simulink model "AGTF30SysDyn"  (R2021b)
settings: Solver=ode4  StartTime=0.0  StopTime=MWS.In.Tsim  FixedStep=MWS.In.Ts  RelTol=1e-3  EnableMultiTasking=on
model workspace: external: MAT-File (data not in the file)
undefined symbols (not defined in the file): MWS, VAFNact, VBVact
libraries: Lib_Cntrl_FirstOrderSensor_TMATS x12, Lib_Cntrl_SetPoint_TMATS x2, Lib_Solve_OuterLoopIntegrator_TMATS x2, simulink x2, Lib_Cntrl_FirstOrderActuator_TMATS x1, Lib_Cntrl_CorrectedSpeed_TMATS x1, Lib_Solve_IterNRSolverJC_TMATS x1
settings Model: Creator=jwchapm2  LastModifiedBy=prbalm
settings SolverCC: AlgebraicLoopSolver=TrustRegion
settings DataIOCC: LimitDataPoints=on  SaveFormat=Array  ReturnWorkspaceOutputs=off
settings OptimizationCC: LifeSpan=inf
settings DebuggingCC: SFUnexpectedBacktrackingDiag=warning  SFNoUnconditionalDefaultTransitionDiag=warning  SFExecutionAtInitializationDiag=none  SFMachineParentedDataDiag=warning  ArithmeticOperatorsInVariantConditions=warning
settings HardwareCC: ProdBitPerPointer=32  ProdBitPerSizeT=32  ProdBitPerPtrDiffT=32  ProdLargestAtomicFloat=None  ProdIntDivRoundTo=Undefined  ProdEndianess=Unspecified  ProdWordSize=32  ProdHWDeviceType=32-bit Generic
settings ModelReferenceCC: PropagateSignalLabelsOutOfModel=off
settings SFSimCC: SimUseLocalCustomCode=off  CustomCodeUndefinedFunction=UseInterfaceOnly
settings RTWCC: RTWUseLocalCustomCode=off
settings CodeAppCC: StateflowObjectComments=on
settings GRTTargetCC: TargetLangStandard=C89/C90 (ANSI)
settings ConfigComp: CovMetricSettings=dw  CovSaveCumulativeToWorkspaceVar=on  CovSaveSingleToWorkspaceVar=on  CovExternalEMLEnable=off

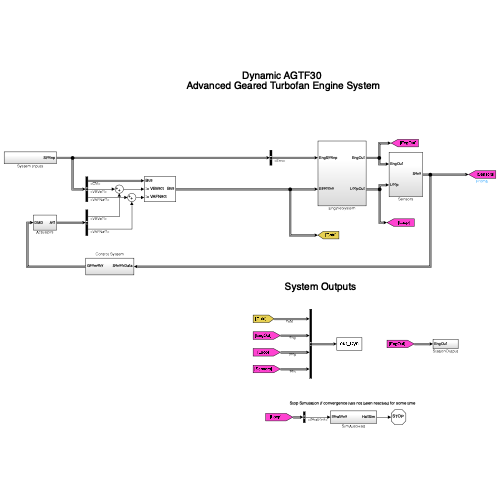
[thumbnail: Simulink's stored preview of the top-level diagram]
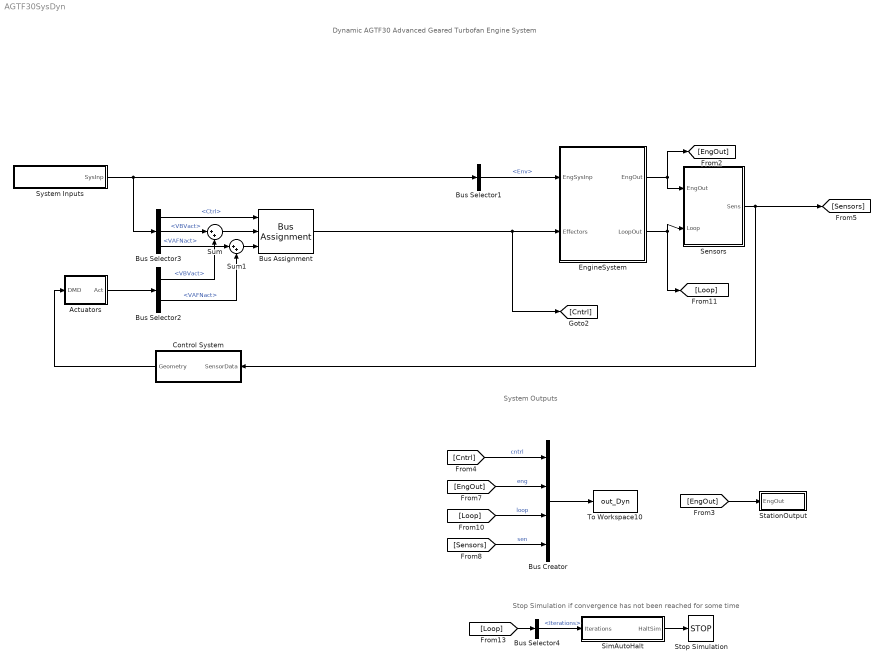
== system AGTF30SysDyn ==
  note: Stop Simulation if convergence has not been reached for some time
  note: Dynamic AGTF30
      | Advanced Geared Turbofan Engine System
  note: System Outputs
  Actuators : Subsystem
  Bus Assignment : BusAssignment  AssignedSignals=VBVact,VAFNact
  Bus Creator : BusCreator  Inputs=4
  Bus Selector1 : BusSelector  OutputSignals=Env
  Bus Selector2 : BusSelector  OutputSignals=VBVact,VAFNact
  Bus Selector3 : BusSelector  OutputSignals=Ctrl,Ctrl.VBVact,Ctrl.VAFNact
  Bus Selector4 : BusSelector  OutputSignals=Solver.Iterations
  Control System : Subsystem
  EngineSystem : Subsystem
  Sensors : Subsystem
  SimAutoHalt : Subsystem
  StationOutput : Subsystem
  Stop Simulation : Stop
  Sum : Sum  Inputs=|++
  Sum1 : Sum  Inputs=|++
  System Inputs : Subsystem
  To Workspace10 : ToWorkspace  VariableName=out_Dyn  SaveFormat=Timeseries  SampleTime=-1
  wires:
  EngineSystem/1(EngOut) -> Sensors/1(EngOut), [EngOut]
  EngineSystem/2(LoopOut) -> Sensors/2(Loop), [Loop]
  [EngOut] -> StationOutput/1(EngOut)
  Bus Creator/1 -> To Workspace10/1
  [Loop] -> Bus Creator/3  "loop"
  [Sensors] -> Bus Creator/4  "sen"
  [EngOut] -> Bus Creator/2  "eng"
  [Cntrl] -> Bus Creator/1  "cntrl"
  [Loop] -> Bus Selector4/1
  Bus Selector4/1 -> SimAutoHalt/1(Iterations)  "<Iterations>"
  SimAutoHalt/1(HaltSim) -> Stop Simulation/1
  Actuators/1(Act) -> Bus Selector2/1
  Control System/1(Geometry) -> Actuators/1(DMD)
  System Inputs/1(SysInp) -> Bus Selector1/1, Bus Selector3/1
  Bus Assignment/1 -> [Cntrl], EngineSystem/2(Effectors)
  Sensors/1(Sens) -> [Sensors], Control System/1(SensorData)
  Bus Selector3/2 -> Sum/1  "<VBVact>"
  Bus Selector2/1 -> Sum/2  "<VBVact>"
  Bus Selector2/2 -> Sum1/2  "<VAFNact>"
  Sum1/1 -> Bus Assignment/3
  Bus Selector1/1 -> EngineSystem/1(EngSysInp)  "<Env>"
  Sum/1 -> Bus Assignment/2
  Bus Selector3/3 -> Sum1/1  "<VAFNact>"
  Bus Selector3/1 -> Bus Assignment/1  "<Ctrl>"

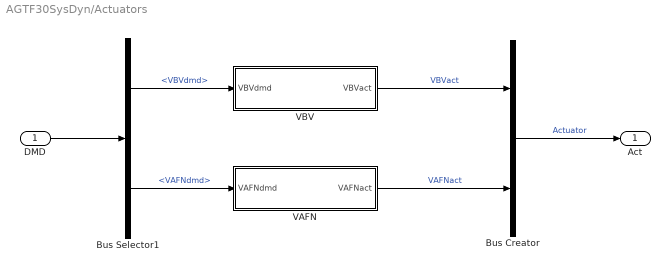
== system AGTF30SysDyn/Actuators ==
  DMD : Inport
  Bus Creator : BusCreator  Inputs=2
  Bus Selector1 : BusSelector  OutputSignals=VBVdmd,VAFNdmd
  VAFN : Subsystem
  VBV : Subsystem
  Act : Outport
  wires:
  DMD/1 -> Bus Selector1/1
  Bus Creator/1 -> Act/1  "Actuator"
  Bus Selector1/2 -> VAFN/1(VAFNdmd)  "<VAFNdmd>"
  Bus Selector1/1 -> VBV/1(VBVdmd)  "<VBVdmd>"
  VBV/1(VBVact) -> Bus Creator/1  "VBVact"
  VAFN/1(VAFNact) -> Bus Creator/2  "VAFNact"

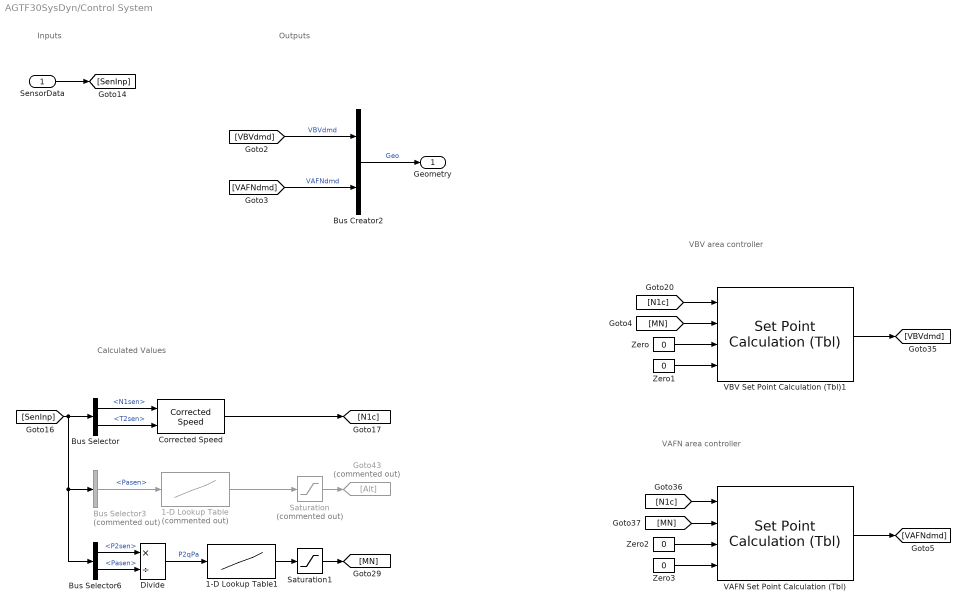
== system AGTF30SysDyn/Control System ==
  note: Inputs
  note: VAFN area controller
  note: VBV area controller
  note: Calculated Values
  note: Outputs
  SensorData : Inport
  1-D Lookup Table : Lookup_n-D  Commented=on  NumberOfTableDimensions=1  BreakpointsForDimension1=MWS.Cntrl.AltCalc_PaVec  Table=MWS.Cntrl.AltCalc_AltVec  InternalRulePriority=Speed  RndMeth=Simplest  InputSameDT=on
  1-D Lookup Table1 : Lookup_n-D  NumberOfTableDimensions=1  BreakpointsForDimension1=MWS.Cntrl.MNCalc_P2qPa  Table=MWS.Cntrl.MNCalc_MNVec  InternalRulePriority=Speed  RndMeth=Simplest  InputSameDT=on
  Bus Creator2 : BusCreator  Inputs=2
  Bus Selector : BusSelector  OutputSignals=N.N1sen,T.T2sen
  Bus Selector3 : BusSelector  Commented=on  OutputSignals=P.Pasen
  Bus Selector6 : BusSelector  OutputSignals=P.P2sen,P.Pasen
  Corrected Speed : Lib_Cntrl_CorrectedSpeed_TMATS/Corrected Speed  C_TSTD_M=518.67
  Divide : Product  Inputs=*/
  Goto43 : Goto  Commented=on  GotoTag=Alt
  Saturation : Saturate  Commented=on  UpperLimit=MWS.Cntrl.AltCalc_Altmax  LowerLimit=MWS.Cntrl.AltCalc_Altmin
  Saturation1 : Saturate  UpperLimit=MWS.Cntrl.MNCalc_MNmax  LowerLimit=MWS.Cntrl.MNCalc_MNmin
  VAFN Set Point Calculation (Tbl) : Lib_Cntrl_SetPoint_TMATS/Set Point Calculation (Tbl)  ERVec_M=MWS.Cntrl.VAFN_Nc1  DSVec_M=MWS.Cntrl.VAFN_MN  SPArray_M=MWS.Cntrl.VAFN_sch
  VBV Set Point Calculation (Tbl)1 : Lib_Cntrl_SetPoint_TMATS/Set Point Calculation (Tbl)  ERVec_M=MWS.Cntrl.VBV_Nc1  DSVec_M=MWS.Cntrl.VBV_MN  SPArray_M=MWS.Cntrl.VBV_sch
  Zero{,1..3} (4 alike) : Constant  Value=0  OutDataTypeStr=Inherit: Inherit via back propagation
  Geometry : Outport
  wires:
  [VBVdmd] -> Bus Creator2/1  "VBVdmd"
  [VAFNdmd] -> Bus Creator2/2  "VAFNdmd"
  SensorData/1 -> [SenInp]
  Bus Selector/1 -> Corrected Speed/1  "<N1sen>"
  Corrected Speed/1 -> [N1c]
  Bus Selector/2 -> Corrected Speed/2  "<T2sen>"
  VAFN Set Point Calculation (Tbl)/1 -> [VAFNdmd]
  [MN] -> VBV Set Point Calculation (Tbl)1/2
  VBV Set Point Calculation (Tbl)1/1 -> [VBVdmd]
  [MN] -> VAFN Set Point Calculation (Tbl)/2
  [N1c] -> VAFN Set Point Calculation (Tbl)/1
  [N1c] -> VBV Set Point Calculation (Tbl)1/1
  1-D Lookup Table/1 -> Saturation/1
  [SenInp] -> Bus Selector6/1, Bus Selector3/1, Bus Selector/1
  Bus Selector3/1 -> 1-D Lookup Table/1  "<Pasen>"
  Bus Selector6/1 -> Divide/1  "<P2sen>"
  Bus Selector6/2 -> Divide/2  "<Pasen>"
  Divide/1 -> 1-D Lookup Table1/1  "P2qPa"
  1-D Lookup Table1/1 -> Saturation1/1
  Saturation/1 -> Goto43/1
  Saturation1/1 -> [MN]
  Bus Creator2/1 -> Geometry/1  "Geo"
  Zero/1 -> VBV Set Point Calculation (Tbl)1/3
  Zero1/1 -> VBV Set Point Calculation (Tbl)1/4
  Zero2/1 -> VAFN Set Point Calculation (Tbl)/3
  Zero3/1 -> VAFN Set Point Calculation (Tbl)/4

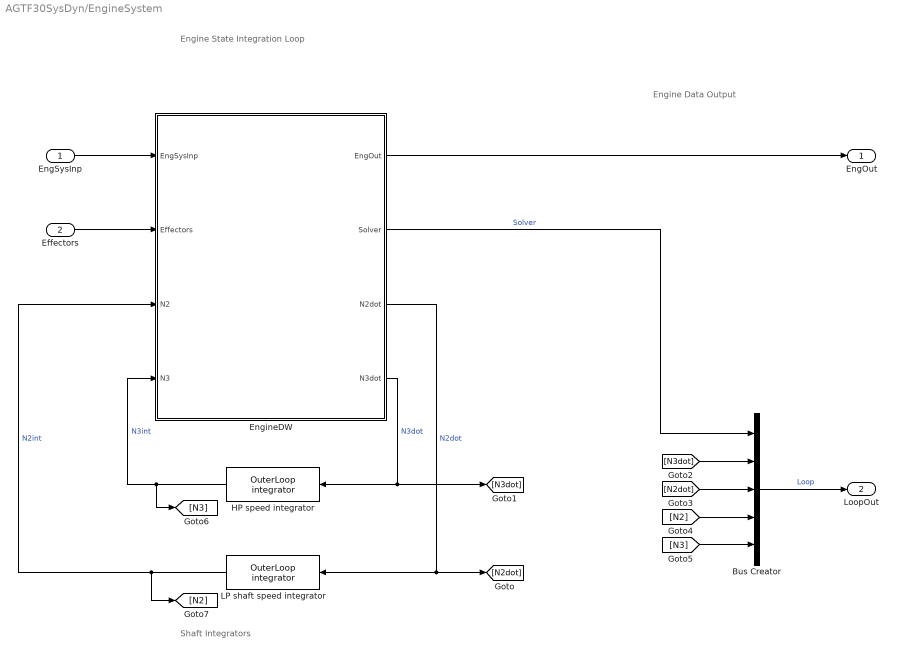
== system AGTF30SysDyn/EngineSystem ==
  note: Shaft Integrators
  note: Engine State
      | Integration Loop
  note: Engine Data Output
  EngSysInp : Inport
  Effectors : Inport  Port=2
  Bus Creator : BusCreator  Inputs=5
  EngineDW : Subsystem
  HP speed integrator : Lib_Solve_OuterLoopIntegrator_TMATS/OuterLoop integrator  OL_IC_M=MWS.In.N3IC
  LP shaft speed integrator : Lib_Solve_OuterLoopIntegrator_TMATS/OuterLoop integrator  OL_IC_M=MWS.In.N2IC
  EngOut : Outport
  LoopOut : Outport  Port=2
  wires:
  EngSysInp/1 -> EngineDW/1(EngSysInp)
  LP shaft speed integrator/1 -> [N2], EngineDW/3(N2)  "N2int"
  Effectors/1 -> EngineDW/2(Effectors)
  EngineDW/3(N2dot) -> LP shaft speed integrator/1, [N2dot]  "N2dot"
  EngineDW/2(Solver) -> Bus Creator/1  "Solver"
  EngineDW/1(EngOut) -> EngOut/1
  EngineDW/4(N3dot) -> HP speed integrator/1, [N3dot]  "N3dot"
  HP speed integrator/1 -> [N3], EngineDW/4(N3)  "N3int"
  Bus Creator/1 -> LoopOut/1  "Loop"
  [N3dot] -> Bus Creator/2
  [N2dot] -> Bus Creator/3
  [N2] -> Bus Creator/4
  [N3] -> Bus Creator/5

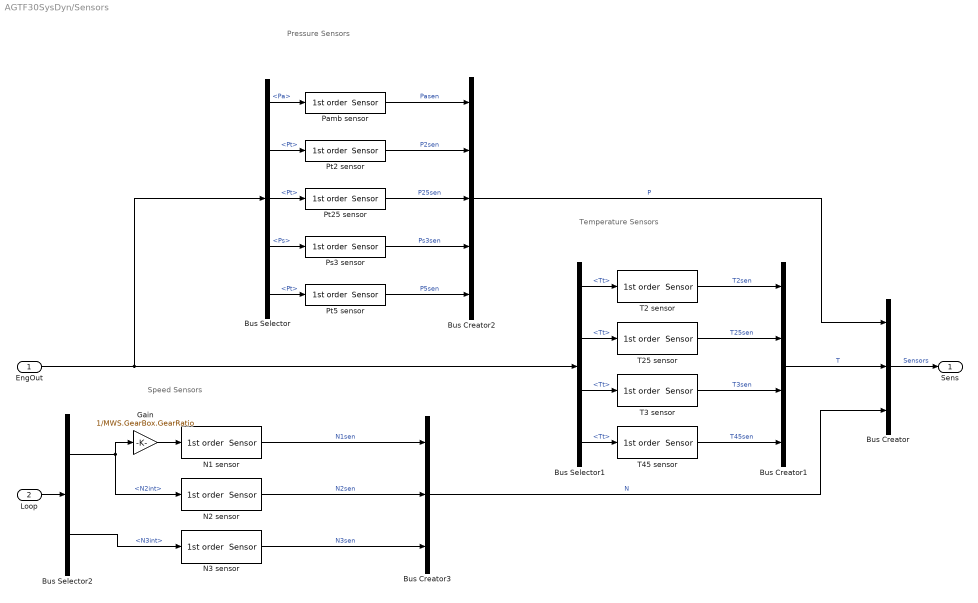
== system AGTF30SysDyn/Sensors ==
  note: Pressure Sensors
  note: Temperature Sensors
  note: Speed Sensors
  EngOut : Inport
  Loop : Inport  Port=2
  Bus Creator : BusCreator  Inputs=3
  Bus Creator1 : BusCreator  Inputs=4
  Bus Creator2 : BusCreator  Inputs=5
  Bus Creator3 : BusCreator  Inputs=3
  Bus Selector : BusSelector  OutputSignals=Amb.Pa,S2.Pt,S25.Pt,S36.Ps,S5.Pt
  Bus Selector1 : BusSelector  OutputSignals=S2.Tt,S25.Tt,S36.Tt,S45.Tt
  Bus Selector2 : BusSelector  OutputSignals=N2int,N3int
  Gain : Gain  Gain=1/MWS.GearBox.GearRatio
  N1 sensor : Lib_Cntrl_FirstOrderSensor_TMATS/1st order  Sensor  IC_M=MWS.In.Sensor.ICN1  Sen_Max_M=MWS.Sensor.N1.Max  Sen_Min_M=MWS.Sensor.N1.Min  Gain_M=1  Tau_M=MWS.Sensor.N1.Tau  GN_EN_M=off  GN_NST_M=MWS.In.Ts  GN_C_M=1  GN_MinNoise_M=0.3  F_Gain_M=1  F_Drift_M=0
  N2 sensor : Lib_Cntrl_FirstOrderSensor_TMATS/1st order  Sensor  IC_M=MWS.In.Sensor.ICN2  Sen_Max_M=MWS.Sensor.N2.Max  Sen_Min_M=MWS.Sensor.N2.Min  Gain_M=1  Tau_M=MWS.Sensor.N2.Tau  GN_EN_M=off  GN_NST_M=MWS.In.Ts  GN_C_M=1  GN_MinNoise_M=0.3  F_Gain_M=1  F_Drift_M=0
  N3 sensor : Lib_Cntrl_FirstOrderSensor_TMATS/1st order  Sensor  IC_M=MWS.In.Sensor.ICN3  Sen_Max_M=MWS.Sensor.N3.Max  Sen_Min_M=MWS.Sensor.N3.Min  Gain_M=1  Tau_M=MWS.Sensor.N3.Tau  GN_EN_M=off  GN_NST_M=MWS.In.Ts  GN_C_M=1  GN_MinNoise_M=0.3  F_Gain_M=1  F_Drift_M=0
  Pamb sensor : Lib_Cntrl_FirstOrderSensor_TMATS/1st order  Sensor  IC_M=MWS.In.Sensor.ICPa  Sen_Max_M=MWS.Sensor.P2.Max  Sen_Min_M=MWS.Sensor.P2.Min  Gain_M=1  Tau_M=MWS.Sensor.P2.Tau  GN_EN_M=off  GN_NST_M=MWS.In.Ts  GN_C_M=1  GN_MinNoise_M=0.3  F_Gain_M=1  F_Drift_M=0
  Ps3 sensor : Lib_Cntrl_FirstOrderSensor_TMATS/1st order  Sensor  IC_M=MWS.In.Sensor.ICPs3  Sen_Max_M=MWS.Sensor.Ps3.Max  Sen_Min_M=MWS.Sensor.Ps3.Min  Gain_M=1  Tau_M=MWS.Sensor.Ps3.Tau  GN_EN_M=off  GN_NST_M=MWS.In.Ts  GN_C_M=1  GN_MinNoise_M=0.3  F_Gain_M=1  F_Drift_M=0
  Pt2 sensor : Lib_Cntrl_FirstOrderSensor_TMATS/1st order  Sensor  IC_M=MWS.In.Sensor.ICP2  Sen_Max_M=MWS.Sensor.P2.Max  Sen_Min_M=MWS.Sensor.P2.Min  Gain_M=1  Tau_M=MWS.Sensor.P2.Tau  GN_EN_M=off  GN_NST_M=MWS.In.Ts  GN_C_M=1  GN_MinNoise_M=0.3  F_Gain_M=1  F_Drift_M=0
  Pt25 sensor : Lib_Cntrl_FirstOrderSensor_TMATS/1st order  Sensor  IC_M=MWS.In.Sensor.ICP25  Sen_Max_M=MWS.Sensor.P25.Max  Sen_Min_M=MWS.Sensor.P25.Min  Gain_M=1  Tau_M=MWS.Sensor.P25.Tau  GN_EN_M=off  GN_NST_M=MWS.In.Ts  GN_C_M=1  GN_MinNoise_M=0.3  F_Gain_M=1  F_Drift_M=0
  Pt5 sensor : Lib_Cntrl_FirstOrderSensor_TMATS/1st order  Sensor  IC_M=MWS.In.Sensor.ICP5  Sen_Max_M=MWS.Sensor.P5.Max  Sen_Min_M=MWS.Sensor.P5.Min  Gain_M=1  Tau_M=MWS.Sensor.P5.Tau  GN_EN_M=off  GN_NST_M=MWS.In.Ts  GN_C_M=1  GN_MinNoise_M=0.3  F_Gain_M=1  F_Drift_M=0
  T2 sensor : Lib_Cntrl_FirstOrderSensor_TMATS/1st order  Sensor  IC_M=MWS.In.Sensor.ICT2  Sen_Max_M=MWS.Sensor.T2.Max  Sen_Min_M=MWS.Sensor.T2.Min  Gain_M=1  Tau_M=MWS.Sensor.T2.Tau  GN_EN_M=off  GN_NST_M=MWS.In.Ts  GN_C_M=1  GN_MinNoise_M=0.3  F_Gain_M=1  F_Drift_M=0
  T25 sensor : Lib_Cntrl_FirstOrderSensor_TMATS/1st order  Sensor  IC_M=MWS.In.Sensor.ICT25  Sen_Max_M=MWS.Sensor.T25.Max  Sen_Min_M=MWS.Sensor.T25.Min  Gain_M=1  Tau_M=MWS.Sensor.T25.Tau  GN_EN_M=off  GN_NST_M=MWS.In.Ts  GN_C_M=1  GN_MinNoise_M=0.3  F_Gain_M=1  F_Drift_M=0
  T3 sensor : Lib_Cntrl_FirstOrderSensor_TMATS/1st order  Sensor  IC_M=MWS.In.Sensor.ICT3  Sen_Max_M=MWS.Sensor.T3.Max  Sen_Min_M=MWS.Sensor.T3.Min  Gain_M=1  Tau_M=MWS.Sensor.T3.Tau  GN_EN_M=off  GN_NST_M=MWS.In.Ts  GN_C_M=1  GN_MinNoise_M=0.3  F_Gain_M=1  F_Drift_M=0
  T45 sensor : Lib_Cntrl_FirstOrderSensor_TMATS/1st order  Sensor  IC_M=MWS.In.Sensor.ICT45  Sen_Max_M=MWS.Sensor.T45.Max*10  Sen_Min_M=MWS.Sensor.T45.Min  Gain_M=1  Tau_M=MWS.Sensor.T45.Tau  GN_EN_M=off  GN_NST_M=MWS.In.Ts  GN_C_M=1  GN_MinNoise_M=0.3  F_Gain_M=1  F_Drift_M=0
  Sens : Outport
  wires:
  Bus Creator/1 -> Sens/1  "Sensors"
  Bus Selector/2 -> Pt2 sensor/1  "<Pt>"
  Bus Creator2/1 -> Bus Creator/1  "P"
  Bus Creator1/1 -> Bus Creator/2  "T"
  Bus Selector1/1 -> T2 sensor/1  "<Tt>"
  Bus Creator3/1 -> Bus Creator/3  "N"
  Bus Selector/3 -> Pt25 sensor/1  "<Pt>"
  Bus Selector/5 -> Pt5 sensor/1  "<Pt>"
  Pt2 sensor/1 -> Bus Creator2/2  "P2sen"
  Pt25 sensor/1 -> Bus Creator2/3  "P25sen"
  Pt5 sensor/1 -> Bus Creator2/5  "P5sen"
  Bus Selector1/2 -> T25 sensor/1  "<Tt>"
  Bus Selector1/3 -> T3 sensor/1  "<Tt>"
  Bus Selector1/4 -> T45 sensor/1  "<Tt>"
  T2 sensor/1 -> Bus Creator1/1  "T2sen"
  T25 sensor/1 -> Bus Creator1/2  "T25sen"
  T3 sensor/1 -> Bus Creator1/3  "T3sen"
  N1 sensor/1 -> Bus Creator3/1  "N1sen"
  Bus Selector/4 -> Ps3 sensor/1  "<Ps>"
  N3 sensor/1 -> Bus Creator3/3  "N3sen"
  Bus Selector/1 -> Pamb sensor/1  "<Pa>"
  Pamb sensor/1 -> Bus Creator2/1  "Pasen"
  N2 sensor/1 -> Bus Creator3/2  "N2sen"
  EngOut/1 -> Bus Selector/1, Bus Selector1/1
  Bus Selector2/2 -> N3 sensor/1  "<N3int>"
  Bus Selector2/1 -> N2 sensor/1, Gain/1  "<N2int>"
  Gain/1 -> N1 sensor/1
  Loop/1 -> Bus Selector2/1
  T45 sensor/1 -> Bus Creator1/4  "T45sen"
  Ps3 sensor/1 -> Bus Creator2/4  "Ps3sen"

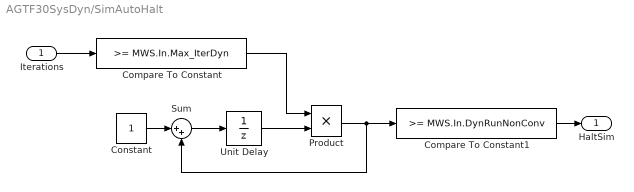
== system AGTF30SysDyn/SimAutoHalt ==
  Iterations : Inport
  Compare To Constant : simulink/Logic and Bit Operations/Compare To Constant  relop=>=  const=MWS.In.Max_IterDyn  OutDataTypeStr=boolean
  Compare To Constant1 : simulink/Logic and Bit Operations/Compare To Constant  relop=>=  const=MWS.In.DynRunNonConv  OutDataTypeStr=boolean
  Constant : Constant
  Product : Product
  Sum : Sum  Inputs=|++
  Unit Delay : UnitDelay  SampleTime=-1  HasFrameUpgradeWarning=on
  HaltSim : Outport
  wires:
  Compare To Constant1/1 -> HaltSim/1
  Iterations/1 -> Compare To Constant/1
  Compare To Constant/1 -> Product/1
  Constant/1 -> Sum/1
  Sum/1 -> Unit Delay/1
  Unit Delay/1 -> Product/2
  Product/1 -> Sum/2, Compare To Constant1/1

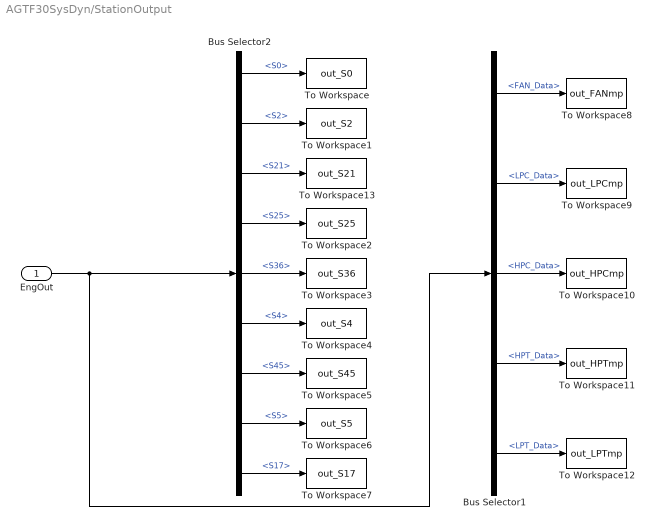
== system AGTF30SysDyn/StationOutput ==
  EngOut : Inport
  Bus Selector1 : BusSelector  OutputSignals=Data.FAN_Data,Data.LPC_Data,Data.HPC_Data,Data.HPT_Data,Data.LPT_Data
  Bus Selector2 : BusSelector  OutputSignals=S0,S2,S21,S25,S36,S4,S45,S5,S17
  To Workspace : ToWorkspace  VariableName=out_S0  SaveFormat=Timeseries  SampleTime=-1
  To Workspace1 : ToWorkspace  VariableName=out_S2  SaveFormat=Timeseries  SampleTime=-1
  To Workspace10 : ToWorkspace  VariableName=out_HPCmp  SaveFormat=Timeseries  SampleTime=-1
  To Workspace11 : ToWorkspace  VariableName=out_HPTmp  SaveFormat=Timeseries  SampleTime=-1
  To Workspace12 : ToWorkspace  VariableName=out_LPTmp  SaveFormat=Timeseries  SampleTime=-1
  To Workspace13 : ToWorkspace  VariableName=out_S21  SaveFormat=Timeseries  SampleTime=-1
  To Workspace2 : ToWorkspace  VariableName=out_S25  SaveFormat=Timeseries  SampleTime=-1
  To Workspace3 : ToWorkspace  VariableName=out_S36  SaveFormat=Timeseries  SampleTime=-1
  To Workspace4 : ToWorkspace  VariableName=out_S4  SaveFormat=Timeseries  SampleTime=-1
  To Workspace5 : ToWorkspace  VariableName=out_S45  SaveFormat=Timeseries  SampleTime=-1
  To Workspace6 : ToWorkspace  VariableName=out_S5  SaveFormat=Timeseries  SampleTime=-1
  To Workspace7 : ToWorkspace  VariableName=out_S17  SaveFormat=Timeseries  SampleTime=-1
  To Workspace8 : ToWorkspace  VariableName=out_FANmp  SaveFormat=Timeseries  SampleTime=-1
  To Workspace9 : ToWorkspace  VariableName=out_LPCmp  SaveFormat=Timeseries  SampleTime=-1
  wires:
  Bus Selector2/3 -> To Workspace13/1  "<S21>"
  Bus Selector2/1 -> To Workspace/1  "<S0>"
  EngOut/1 -> Bus Selector1/1, Bus Selector2/1
  Bus Selector2/2 -> To Workspace1/1  "<S2>"
  Bus Selector2/4 -> To Workspace2/1  "<S25>"
  Bus Selector2/5 -> To Workspace3/1  "<S36>"
  Bus Selector2/6 -> To Workspace4/1  "<S4>"
  Bus Selector2/7 -> To Workspace5/1  "<S45>"
  Bus Selector2/8 -> To Workspace6/1  "<S5>"
  Bus Selector2/9 -> To Workspace7/1  "<S17>"
  Bus Selector1/1 -> To Workspace8/1  "<FAN_Data>"
  Bus Selector1/2 -> To Workspace9/1  "<LPC_Data>"
  Bus Selector1/3 -> To Workspace10/1  "<HPC_Data>"
  Bus Selector1/4 -> To Workspace11/1  "<HPT_Data>"
  Bus Selector1/5 -> To Workspace12/1  "<LPT_Data>"

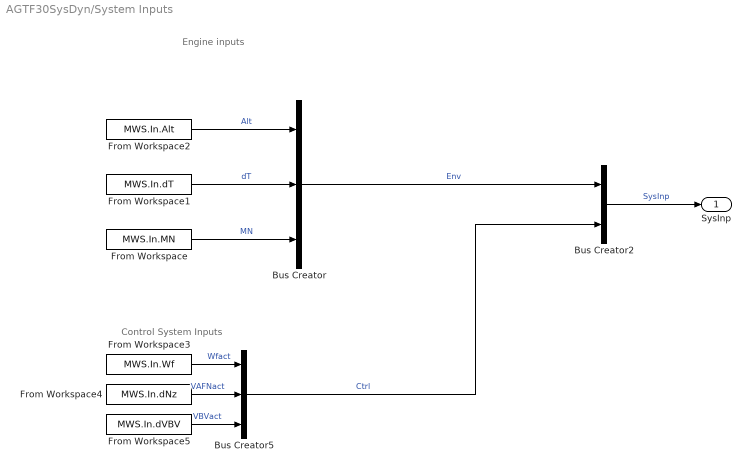
== system AGTF30SysDyn/System Inputs ==
  note: Engine inputs
  note: Control System Inputs
  Bus Creator : BusCreator  Inputs=3
  Bus Creator2 : BusCreator  Inputs=2
  Bus Creator5 : BusCreator  Inputs=3
  From Workspace : FromWorkspace  VariableName=MWS.In.MN
  From Workspace1 : FromWorkspace  VariableName=MWS.In.dT
  From Workspace2 : FromWorkspace  VariableName=MWS.In.Alt
  From Workspace3 : FromWorkspace  VariableName=MWS.In.Wf
  From Workspace4 : FromWorkspace  VariableName=MWS.In.dNz
  From Workspace5 : FromWorkspace  VariableName=MWS.In.dVBV
  SysInp : Outport
  wires:
  From Workspace2/1 -> Bus Creator/1  "Alt"
  From Workspace1/1 -> Bus Creator/2  "dT"
  From Workspace/1 -> Bus Creator/3  "MN"
  Bus Creator/1 -> Bus Creator2/1  "Env"
  Bus Creator5/1 -> Bus Creator2/2  "Ctrl"
  Bus Creator2/1 -> SysInp/1  "SysInp"
  From Workspace3/1 -> Bus Creator5/1  "Wfact"
  From Workspace4/1 -> Bus Creator5/2  "VAFNact"
  From Workspace5/1 -> Bus Creator5/3  "VBVact"

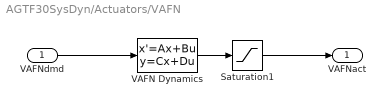
== system AGTF30SysDyn/Actuators/VAFN ==
  VAFNdmd : Inport
  Saturation1 : Saturate  UpperLimit=MWS.Act.VAFN_max  LowerLimit=0  LinearizeAsGain=off
  VAFN Dynamics : StateSpace  A=MWS.Act.VAFN.A  B=MWS.Act.VAFN.B  C=MWS.Act.VAFN.C  D=MWS.Act.VAFN.D  InitialCondition=MWS.In.VAFNIC
  VAFNact : Outport
  wires:
  Saturation1/1 -> VAFNact/1
  VAFNdmd/1 -> VAFN Dynamics/1
  VAFN Dynamics/1 -> Saturation1/1

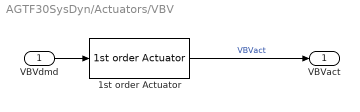
== system AGTF30SysDyn/Actuators/VBV ==
  VBVdmd : Inport
  1st order Actuator : Lib_Cntrl_FirstOrderActuator_TMATS/1st order Actuator  Gain_M=MWS.Act.VBV.Gain  Tau_M=MWS.Act.VBV.Tau  IC_M=MWS.In.VBVIC  MaxSat_M=MWS.Act.VBV.max  MinSat_M=MWS.Act.VBV.min  deadband_M=0.0  rateLimit_M=100000
  VBVact : Outport
  wires:
  VBVdmd/1 -> 1st order Actuator/1
  1st order Actuator/1 -> VBVact/1  "VBVact"

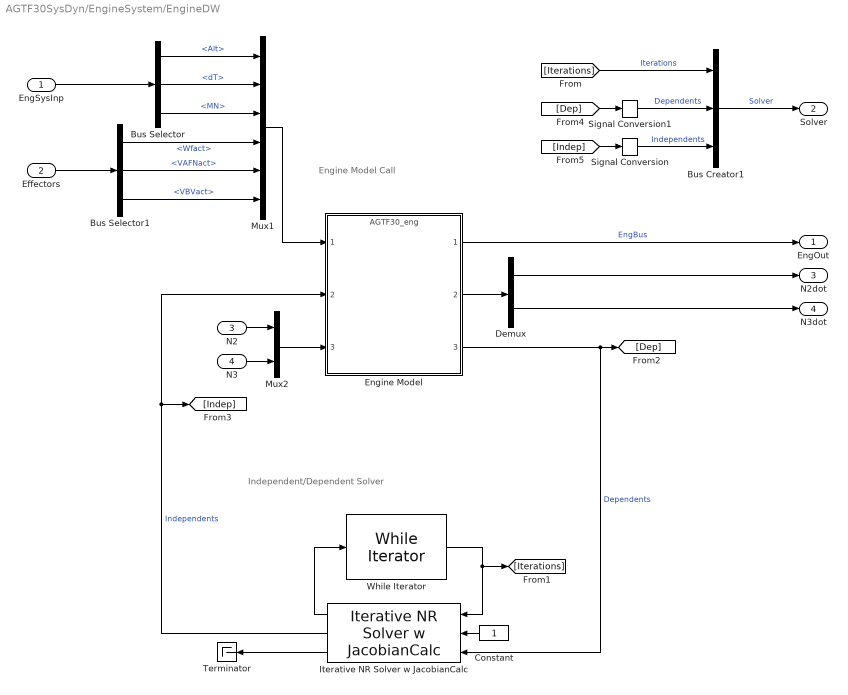
== system AGTF30SysDyn/EngineSystem/EngineDW ==
  note: Independent/Dependent Solver
  note: Engine Model Call
  EngSysInp : Inport
  Effectors : Inport  Port=2
  N2 : Inport  Port=3
  N3 : Inport  Port=4
  Bus Creator1 : BusCreator  Inputs=3
  Bus Selector : BusSelector  OutputSignals=Alt,dT,MN
  Bus Selector1 : BusSelector  OutputSignals=Wfact,VAFNact,VBVact
  Constant : Constant
  Demux : Demux  Outputs=2
  Engine Model : ModelReference  ModelNameDialog=AGTF30_eng.mdl  SimulationMode=Normal  ModelReferenceVersion=1.306
  Iterative NR Solver w JacobianCalc : Lib_Solve_IterNRSolverJC_TMATS/Iterative NR Solver w JacobianCalc  SJac_Per_M=MWS.In.JPerDyn  SNR_IC_M=MWS.In.ICcom  SNR_DX_M=MWS.In.dX  SNR_Mx_M=100000  SNR_Mn_M=0.0001  SJacobianAttempts_M=MWS.In.NRADyn  Cond_Limits_M=MWS.In.Lim
  Mux1 : Mux  Inputs=6
  Mux2 : Mux  Inputs=2
  Signal Conversion : SignalConversion  OverrideOpt=off
  Signal Conversion1 : SignalConversion  OverrideOpt=off
  Terminator : Terminator
  While Iterator : WhileIterator  MaxIters=MWS.In.Max_IterDyn  WhileBlockType=do-while  ShowIterationPort=on
  EngOut : Outport
  Solver : Outport  Port=2
  N2dot : Outport  Port=3
  N3dot : Outport  Port=4
  wires:
  Engine Model/1 -> EngOut/1  "EngBus"
  Mux1/1 -> Engine Model/1
  Effectors/1 -> Bus Selector1/1
  Constant/1 -> Iterative NR Solver w JacobianCalc/2
  Iterative NR Solver w JacobianCalc/2 -> Engine Model/2, [Indep]  "Independents"
  Engine Model/3 -> Iterative NR Solver w JacobianCalc/3, [Dep]  "Dependents"
  While Iterator/1 -> [Iterations], Iterative NR Solver w JacobianCalc/1
  Iterative NR Solver w JacobianCalc/1 -> While Iterator/1
  Engine Model/2 -> Demux/1
  Mux2/1 -> Engine Model/3
  Iterative NR Solver w JacobianCalc/3 -> Terminator/1
  N2/1 -> Mux2/1
  N3/1 -> Mux2/2
  Demux/1 -> N2dot/1
  Demux/2 -> N3dot/1
  Bus Selector/1 -> Mux1/1  "<Alt>"
  Bus Selector/2 -> Mux1/2  "<dT>"
  Bus Selector/3 -> Mux1/3  "<MN>"
  Bus Selector1/3 -> Mux1/6  "<VBVact>"
  Bus Selector1/1 -> Mux1/4  "<Wfact>"
  [Iterations] -> Bus Creator1/1  "Iterations"
  Bus Creator1/1 -> Solver/1  "Solver"
  [Dep] -> Signal Conversion1/1
  [Indep] -> Signal Conversion/1
  Signal Conversion/1 -> Bus Creator1/3  "Independents"
  Signal Conversion1/1 -> Bus Creator1/2  "Dependents"
  Bus Selector1/2 -> Mux1/5  "<VAFNact>"
  EngSysInp/1 -> Bus Selector/1
